simulink model "model8"  (R2014a)
settings: Solver=ode4  SolverMode=SingleTasking  StartTime=0.0  StopTime=200.0  FixedStep=.1  RelTol=1e-3
values from neighbouring files (symbols this model uses):
  K0 = diag([w^3,w^3,w^3.5])    [robot_mod_run.m]
  K1 = diag([2*w,2*w,4*w])    [robot_mod_run.m]
  k_ts = 0.29    [robot_mod_run.m]
  Kd = diag([5.4, 5.5, 3.8])    [robot_mod_run.m]
  Kp = diag([1, 1, 1])    [robot_mod_run.m]
  l_ts = .95    (= 0.95)    [robot_mod_run.m]
  qd1 = 1    [robot_mod_run.m]
  qd2 = 1    [robot_mod_run.m]
  qd3 = 1    [robot_mod_run.m]
  R_ts = .5    (= 0.5)    [robot_mod_run.m]
  time_gain_ts = .278    (= 0.278)    [robot_mod_run.m]
undefined symbols (not defined in the file or in its folder): forward_optim
libraries: aerolibutil x3
settings Model: Creator=Fu  LastModifiedBy=Fu
settings OptimizationCC: BlockReduction=off  BooleanDataType=off
settings DebuggingCC: SaveWithParameterizedLinksMsg=none  UnderspecifiedInitializationDetection=Classic  SignalResolutionControl=TryResolveAllWithWarning  SolverPrmCheckMsg=none
settings HardwareCC: TargetUnknown=on

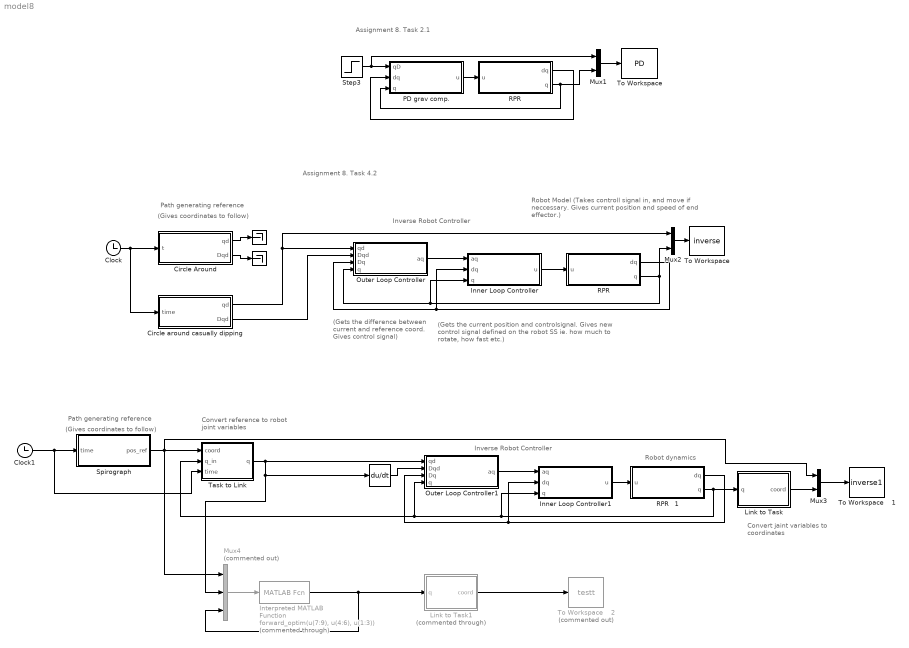
== system model8 ==
  note: Convert jaint variables
      | to coordinates
  note: Robot dynamics
  note: Convert reference to
      | robot joint variables
  note: (Gets the current position and controlsignal.
      | Gives new control signal defined on the robot SS
      | ie. how much to rotate, how fast etc.)
  note: (Gets the difference between
      |  current and reference coord.
      | Gives control signal)
  note: (Gives coordinates to follow)
  note: Robot Model
      | (Takes controll signal in, and move if neccessary.
      | Gives current position and speed of end effector.)
  note: Inverse Robot Controller
  note: Path generating reference
  note: Assignment 8. Task 4.2
  note: Assignment 8. Task 2.1
  note: Inverse Robot Controller
  note: (Gives coordinates to follow)
  note: Path generating reference
  " " : Derivative
  " " : Terminator
  "  " : Terminator
  Circle Around : Subsystem
  Circle around casually dipping : Subsystem
  Clock : Clock
  Clock1 : Clock
  Inner Loop Controller : Subsystem
  Inner Loop Controller1 : Subsystem
  Interpreted MATLAB Function : MATLABFcn  Commented=through  MATLABFcn=forward_optim(u(7:9), u(4:6), u(1:3))  OutputDimensions=3
  Link to Task : MATLAB Function  TreatAsAtomicUnit=on
  Link to Task1 : MATLAB Function  Commented=through  TreatAsAtomicUnit=on
  Mux1 : Mux  Inputs=2
  Mux2 : Mux  Inputs=2
  Mux3 : Mux  Inputs=2
  Mux4 : Mux  Commented=on  Inputs=3
  Outer Loop Controller : Subsystem
  Outer Loop Controller1 : Subsystem
  PD grav comp. : Subsystem
  RPR : Subsystem
  "RPR   " : Subsystem
  RPR   1 : Subsystem
  "Spirograph " : Subsystem
  Step3 : Step  Time=0  Before=[0;0;0]  After=[qd1;qd2;qd3]  SampleTime=0
  Task to Link : MATLAB Function  TreatAsAtomicUnit=on
  To Workspace : ToWorkspace  VariableName=PD  SaveFormat=Timeseries  SampleTime=-1
      settings: Save2DSignal=2-D array (concatenate along first dimension)
  "To Workspace    " : ToWorkspace  VariableName=inverse  SaveFormat=Timeseries  SampleTime=-1
      settings: Save2DSignal=2-D array (concatenate along first dimension)
  To Workspace    1 : ToWorkspace  VariableName=inverse1  SaveFormat=Timeseries  SampleTime=-1
      settings: Save2DSignal=2-D array (concatenate along first dimension)
  To Workspace    2 : ToWorkspace  Commented=on  VariableName=testt  SaveFormat=Timeseries  SampleTime=-1
      settings: Save2DSignal=2-D array (concatenate along first dimension)
  wires:
  PD grav comp./1(u) -> RPR/1(u)
  Step3/1 -> Mux1/1, PD grav comp./1(qD)
  RPR/2(q) -> Mux1/2, PD grav comp./3(q)
  RPR/1(dq) -> PD grav comp./2(dq)
  Inner Loop Controller/1(u) -> "RPR   "/1(u)
  "RPR   "/2(q) -> Mux2/2, Inner Loop Controller/3(q), Outer Loop Controller/4(q)
  "RPR   "/1(dq) -> Outer Loop Controller/3(Dq), Inner Loop Controller/2(dq)
  Outer Loop Controller/1(aq) -> Inner Loop Controller/1(aq)
  Clock/1 -> Circle around casually dipping/1(time), Circle Around/1(t)
  Mux1/1 -> To Workspace/1
  Mux2/1 -> "To Workspace    "/1
  Circle around casually dipping/1(qd) -> Outer Loop Controller/1(qd), Mux2/1
  Circle around casually dipping/2(Dqd) -> Outer Loop Controller/2(Dqd)
  Circle Around/1(qd) -> " "/1
  Circle Around/2(Dqd) -> "  "/1
  Inner Loop Controller1/1(u) -> RPR   1/1(u)
  RPR   1/2(q) -> Link to Task/1(q), Inner Loop Controller1/3(q), Outer Loop Controller1/4(q), Task to Link/2(q_in)
  RPR   1/1(dq) -> Outer Loop Controller1/3(Dq), Inner Loop Controller1/2(dq)
  Outer Loop Controller1/1(aq) -> Inner Loop Controller1/1(aq)
  Clock1/1 -> Task to Link/3(time), "Spirograph "/1(time)
  "Spirograph "/1(pos_ref) -> Mux4/1, Mux3/1, Task to Link/1(coord)
  Task to Link/1(q) -> Outer Loop Controller1/1(qd), " "/1, Mux4/2
  " "/1 -> Outer Loop Controller1/2(Dqd)
  Mux3/1 -> To Workspace    1/1
  Link to Task/1(coord) -> Mux3/2
  Mux4/1 -> Interpreted MATLAB Function/1
  Interpreted MATLAB Function/1 -> Mux4/3, Link to Task1/1(q)
  Link to Task1/1(coord) -> To Workspace    2/1

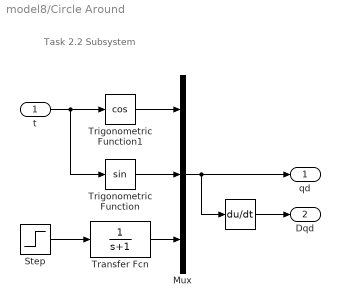
== system model8/Circle Around ==
  note: Task 2.2 Subsystem
  t : Inport
  " " : Derivative
  Mux : Mux  Inputs=3
  Step : Step  SampleTime=0
  Transfer Fcn : TransferFcn  Denominator=[1 1]
  Trigonometric Function : Trigonometry
  Trigonometric Function1 : Trigonometry  Operator=cos
  qd : Outport
  Dqd : Outport  Port=2
  wires:
  Mux/1 -> " "/1, qd/1
  t/1 -> Trigonometric Function/1, Trigonometric Function1/1
  Trigonometric Function1/1 -> Mux/1
  Trigonometric Function/1 -> Mux/2
  Step/1 -> Transfer Fcn/1
  Transfer Fcn/1 -> Mux/3
  " "/1 -> Dqd/1

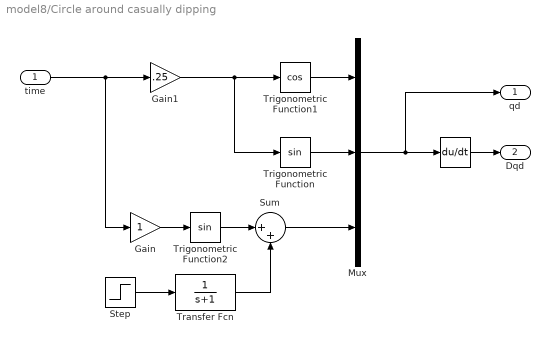
== system model8/Circle around casually dipping ==
  time : Inport
  " " : Derivative
  Gain : Gain
  Gain1 : Gain  Gain=.25
  Mux : Mux  Inputs=3
  Step : Step  SampleTime=0
  Sum : Sum  Inputs=|++
  Transfer Fcn : TransferFcn  Denominator=[1 1]
  Trigonometric Function : Trigonometry
  Trigonometric Function1 : Trigonometry  Operator=cos
  Trigonometric Function2 : Trigonometry
  qd : Outport
  Dqd : Outport  Port=2
  wires:
  Trigonometric Function1/1 -> Mux/1
  Trigonometric Function/1 -> Mux/2
  Mux/1 -> " "/1, qd/1
  " "/1 -> Dqd/1
  time/1 -> Gain1/1, Gain/1
  Step/1 -> Transfer Fcn/1
  Sum/1 -> Mux/3
  Transfer Fcn/1 -> Sum/2
  Gain/1 -> Trigonometric Function2/1
  Trigonometric Function2/1 -> Sum/1
  Gain1/1 -> Trigonometric Function1/1, Trigonometric Function/1

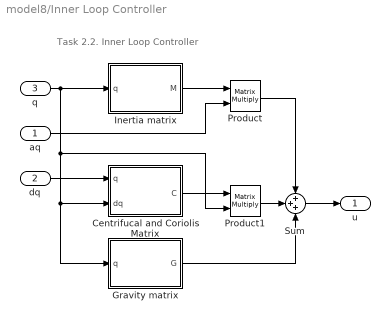
== system model8/Inner Loop Controller ==
  note: Task 2.2. Inner Loop Controller
  aq : Inport
  dq : Inport  Port=2
  q : Inport  Port=3
  Centrifucal and Coriolis Matrix : MATLAB Function  TreatAsAtomicUnit=on
  Gravity matrix : MATLAB Function  TreatAsAtomicUnit=on
  Inertia matrix : MATLAB Function  TreatAsAtomicUnit=on
  Product : Product  Multiplication=Matrix(*)
  Product1 : Product  Multiplication=Matrix(*)
  Sum : Sum  Inputs=+++
  u : Outport
  wires:
  Inertia matrix/1(M) -> Product/1
  aq/1 -> Product/2
  q/1 -> Inertia matrix/1(q), Centrifucal and Coriolis Matrix/2(dq), Gravity matrix/1(q), Product1/2
  Product/1 -> Sum/1
  dq/1 -> Centrifucal and Coriolis Matrix/1(q)
  Centrifucal and Coriolis Matrix/1(C) -> Product1/1
  Product1/1 -> Sum/2
  Gravity matrix/1(G) -> Sum/3
  Sum/1 -> u/1

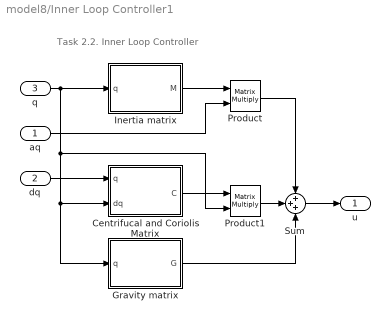
== system model8/Inner Loop Controller1 ==
  note: Task 2.2. Inner Loop Controller
  aq : Inport
  dq : Inport  Port=2
  q : Inport  Port=3
  Centrifucal and Coriolis Matrix : MATLAB Function  TreatAsAtomicUnit=on
  Gravity matrix : MATLAB Function  TreatAsAtomicUnit=on
  Inertia matrix : MATLAB Function  TreatAsAtomicUnit=on
  Product : Product  Multiplication=Matrix(*)
  Product1 : Product  Multiplication=Matrix(*)
  Sum : Sum  Inputs=+++
  u : Outport
  wires:
  Inertia matrix/1(M) -> Product/1
  aq/1 -> Product/2
  q/1 -> Inertia matrix/1(q), Centrifucal and Coriolis Matrix/2(dq), Gravity matrix/1(q), Product1/2
  Product/1 -> Sum/1
  dq/1 -> Centrifucal and Coriolis Matrix/1(q)
  Centrifucal and Coriolis Matrix/1(C) -> Product1/1
  Product1/1 -> Sum/2
  Gravity matrix/1(G) -> Sum/3
  Sum/1 -> u/1

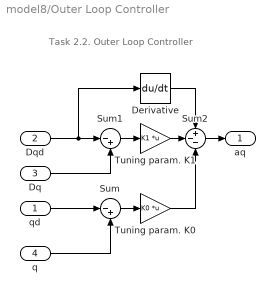
== system model8/Outer Loop Controller ==
  note: Task 2.2. Outer Loop Controller
  qd : Inport
  Dqd : Inport  Port=2
  Dq : Inport  Port=3
  q : Inport  Port=4
  Derivative : Derivative
  Sum : Sum  Inputs=|-+
  Sum1 : Sum  Inputs=|-+
  Sum2 : Sum  Inputs=+--
  Tuning param. K0 : Gain  Gain=K0  Multiplication=Matrix(K*u) (u vector)
  Tuning param. K1 : Gain  Gain=K1  Multiplication=Matrix(K*u) (u vector)
  aq : Outport
  wires:
  qd/1 -> Sum/1
  q/1 -> Sum/2
  Dq/1 -> Sum1/2
  Sum2/1 -> aq/1
  Derivative/1 -> Sum2/1
  Dqd/1 -> Derivative/1, Sum1/1
  Tuning param. K1/1 -> Sum2/2
  Sum1/1 -> Tuning param. K1/1
  Sum/1 -> Tuning param. K0/1
  Tuning param. K0/1 -> Sum2/3

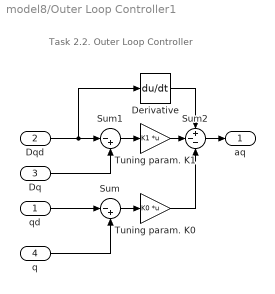
== system model8/Outer Loop Controller1 ==
  note: Task 2.2. Outer Loop Controller
  qd : Inport
  Dqd : Inport  Port=2
  Dq : Inport  Port=3
  q : Inport  Port=4
  Derivative : Derivative
  Sum : Sum  Inputs=|-+
  Sum1 : Sum  Inputs=|-+
  Sum2 : Sum  Inputs=+--
  Tuning param. K0 : Gain  Gain=K0  Multiplication=Matrix(K*u) (u vector)
  Tuning param. K1 : Gain  Gain=K1  Multiplication=Matrix(K*u) (u vector)
  aq : Outport
  wires:
  qd/1 -> Sum/1
  q/1 -> Sum/2
  Dq/1 -> Sum1/2
  Sum2/1 -> aq/1
  Derivative/1 -> Sum2/1
  Dqd/1 -> Derivative/1, Sum1/1
  Tuning param. K1/1 -> Sum2/2
  Sum1/1 -> Tuning param. K1/1
  Sum/1 -> Tuning param. K0/1
  Tuning param. K0/1 -> Sum2/3

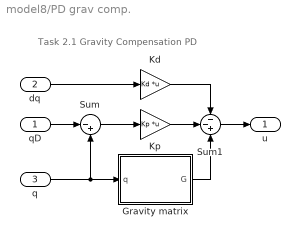
== system model8/PD grav comp. ==
  note: Task 2.1 Gravity Compensation PD
  qD : Inport
  dq : Inport  Port=2
  q : Inport  Port=3
  Gravity matrix : MATLAB Function  TreatAsAtomicUnit=on
  Kd : Gain  Gain=Kd  Multiplication=Matrix(K*u)
  Kp : Gain  Gain=Kp  Multiplication=Matrix(K*u)
  Sum : Sum  Inputs=|-+
  Sum1 : Sum  Inputs=--+
  u : Outport
  wires:
  Sum/1 -> Kp/1
  Kp/1 -> Sum1/2
  Kd/1 -> Sum1/1
  Gravity matrix/1(G) -> Sum1/3
  Sum1/1 -> u/1
  dq/1 -> Kd/1
  q/1 -> Gravity matrix/1(q), Sum/2
  qD/1 -> Sum/1

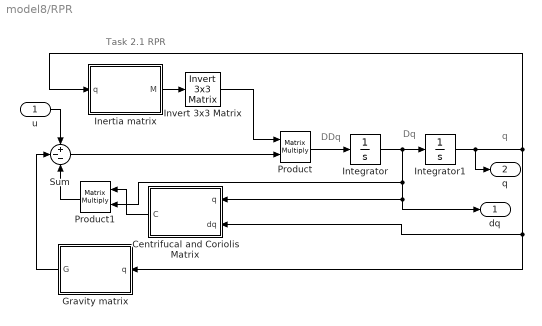
== system model8/RPR ==
  note: Task 2.1 RPR
  note: DDq
  note: q
  note: Dq
  u : Inport
  Centrifucal and Coriolis Matrix : MATLAB Function  TreatAsAtomicUnit=on
  Gravity matrix : MATLAB Function  TreatAsAtomicUnit=on
  Inertia matrix : MATLAB Function  TreatAsAtomicUnit=on
  Integrator : Integrator  InitialCondition=[0;0;0]
  Integrator1 : Integrator  InitialCondition=[1;0;0]
  Invert 3x3 Matrix : aerolibutil/Invert  3x3 Matrix
  Product : Product  Multiplication=Matrix(*)
  Product1 : Product  Multiplication=Matrix(*)
  Sum : Sum  Inputs=+--
  dq : Outport
  q : Outport  Port=2
  wires:
  Inertia matrix/1(M) -> Invert 3x3 Matrix/1
  Invert 3x3 Matrix/1 -> Product/1
  Product/1 -> Integrator/1
  Integrator/1 -> dq/1, Centrifucal and Coriolis Matrix/1(q), Product1/2, Integrator1/1
  Integrator1/1 -> Inertia matrix/1(q), Centrifucal and Coriolis Matrix/2(dq), Gravity matrix/1(q), q/1
  Sum/1 -> Product/2
  u/1 -> Sum/1
  Centrifucal and Coriolis Matrix/1(C) -> Product1/1
  Product1/1 -> Sum/3
  Gravity matrix/1(G) -> Sum/2

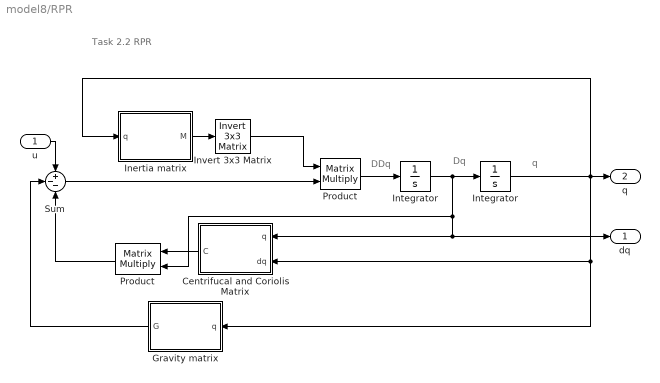
== system model8/RPR    ==
  note: Task 2.2 RPR
  note: DDq
  note: q
  note: Dq
  u : Inport
  Centrifucal and Coriolis Matrix : MATLAB Function  TreatAsAtomicUnit=on
  Gravity matrix : MATLAB Function  TreatAsAtomicUnit=on
  Inertia matrix : MATLAB Function  TreatAsAtomicUnit=on
  Integrator : Integrator  InitialCondition=[0;0;0]
  "Integrator " : Integrator  InitialCondition=[1;0;0]
  Invert 3x3 Matrix : aerolibutil/Invert  3x3 Matrix
  Product : Product  Multiplication=Matrix(*)
  "Product " : Product  Multiplication=Matrix(*)
  Sum : Sum  Inputs=+--
  dq : Outport
  q : Outport  Port=2
  wires:
  Inertia matrix/1(M) -> Invert 3x3 Matrix/1
  Invert 3x3 Matrix/1 -> Product/1
  Product/1 -> Integrator/1
  Integrator/1 -> Centrifucal and Coriolis Matrix/1(q), dq/1, "Product "/2, "Integrator "/1
  "Integrator "/1 -> Inertia matrix/1(q), q/1, Centrifucal and Coriolis Matrix/2(dq), Gravity matrix/1(q)
  Sum/1 -> Product/2
  u/1 -> Sum/1
  Centrifucal and Coriolis Matrix/1(C) -> "Product "/1
  "Product "/1 -> Sum/3
  Gravity matrix/1(G) -> Sum/2

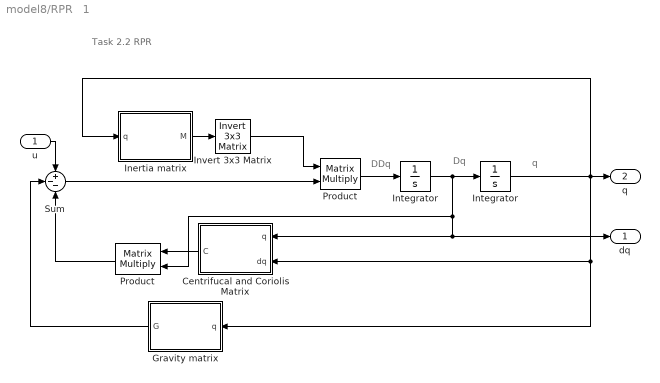
== system model8/RPR   1 ==
  note: Task 2.2 RPR
  note: DDq
  note: q
  note: Dq
  u : Inport
  Centrifucal and Coriolis Matrix : MATLAB Function  TreatAsAtomicUnit=on
  Gravity matrix : MATLAB Function  TreatAsAtomicUnit=on
  Inertia matrix : MATLAB Function  TreatAsAtomicUnit=on
  Integrator : Integrator  InitialCondition=[0;0;0]
  "Integrator " : Integrator  InitialCondition=[0;0;0]
  Invert 3x3 Matrix : aerolibutil/Invert  3x3 Matrix
  Product : Product  Multiplication=Matrix(*)
  "Product " : Product  Multiplication=Matrix(*)
  Sum : Sum  Inputs=+--
  dq : Outport
  q : Outport  Port=2
  wires:
  Inertia matrix/1(M) -> Invert 3x3 Matrix/1
  Invert 3x3 Matrix/1 -> Product/1
  Product/1 -> Integrator/1
  Integrator/1 -> Centrifucal and Coriolis Matrix/1(q), dq/1, "Product "/2, "Integrator "/1
  "Integrator "/1 -> Inertia matrix/1(q), q/1, Centrifucal and Coriolis Matrix/2(dq), Gravity matrix/1(q)
  Sum/1 -> Product/2
  u/1 -> Sum/1
  Centrifucal and Coriolis Matrix/1(C) -> "Product "/1
  "Product "/1 -> Sum/3
  Gravity matrix/1(G) -> Sum/2

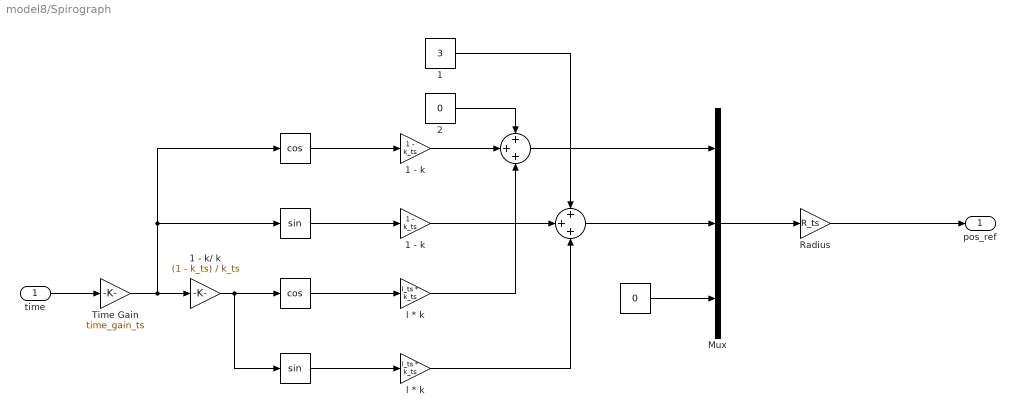
== system model8/Spirograph  ==
  time : Inport
  "    " : Constant  Value=0
  "     " : Trigonometry  Operator=cos
  "      " : Trigonometry
  "       " : Trigonometry  Operator=cos
  "        " : Trigonometry
  "         " : Sum  Inputs=+++
  "          " : Sum  Inputs=+++
  "    1" : Constant  Value=3
  "    2" : Constant  Value=0
  1 - k : Gain  Gain=1 - k_ts
  "1 - k " : Gain  Gain=1 - k_ts
  1 - k/ k : Gain  Gain=(1 - k_ts) / k_ts
  Mux : Mux  Inputs=3
  Radius : Gain  Gain=R_ts
  Time Gain : Gain  Gain=time_gain_ts
  l * k : Gain  Gain=l_ts * k_ts
  "l * k " : Gain  Gain=l_ts * k_ts
  pos_ref : Outport
  wires:
  Mux/1 -> Radius/1
  time/1 -> Time Gain/1
  1 - k/ k/1 -> "       "/1, "        "/1
  "     "/1 -> "1 - k "/1
  "      "/1 -> 1 - k/1
  "       "/1 -> l * k/1
  "        "/1 -> "l * k "/1
  Radius/1 -> pos_ref/1
  Time Gain/1 -> "     "/1, "      "/1, 1 - k/ k/1
  "    "/1 -> Mux/3
  "          "/1 -> Mux/2
  "         "/1 -> Mux/1
  "1 - k "/1 -> "         "/2
  l * k/1 -> "         "/3
  "l * k "/1 -> "          "/3
  1 - k/1 -> "          "/2
  "    1"/1 -> "          "/1
  "    2"/1 -> "         "/1

== matlab function model8/Inner Loop Controller1/Centrifucal and Coriolis Matrix ==
  data: q input; C output; dq input
function C = centriCori(q,dq)
%% Parameters
% Global variables in MATLAB if preferred (remove comments in that case)
% global m1 m2 m3;            % Masses
% global l1 l2 l3;            % Link lengths
% global lc1 lc2 lc3; 	      % Centers of mass
% global In1yy In2zz In3zz;   % Moment of inertia
% global gy;                  % Gravity force

% State variables
q1 = q(1);
q2 = q(2);
q3 = q(3);

dq1 = dq(1);
dq2 = dq(2);
dq3 = dq(3);

%syms q1 q2 q3 dq1 dq2 dq3;
m1 = 5; m2 = 5; m3 = 5;
l1 = 0.5; l2 = 0.5; l3 = 0.5;
lc1 = 0.5/2; lc2 = -0.5/2; lc3 = 0.5/2;
In1yy = 1/12*(m1*(l1)^2);
In2zz = 1/12*(m2*(l2)^2);
In3zz = 1/12*(m3*(l3)^2);

gy =9.81;

%% Matrices
% (8.21) Page 295 in book: M(q)*DDq + C(q,Dq)*Dq + G(q) = u
% Centrifugal and Coriolis matrix
C = [...
        (-0.2e1 * m3 * lc3 * cos(q1) * sin(q1 + q3) + 0.2e1 * m3 * lc3 * sin(q1) * cos(q1 + q3) + 0.2e1 * (m2 + m3) * q2 - 0.2e1 * m2 * lc2) * dq2 / 0.2e1 + (-0.2e1 * m3 * lc3 * cos(q1) * q2 * cos(q1 + q3) - 0.2e1 * m3 * lc3 * sin(q1) * q2 * sin(q1 + q3)) * dq3 / 0.2e1 (-0.2e1 * m3 * lc3 * cos(q1) * sin(q1 + q3) + 0.2e1 * m3 * lc3 * sin(q1) * cos(q1 + q3) + 0.2e1 * (m2 + m3) * q2 - 0.2e1 * m2 * lc2) * dq1 / 0.2e1 (-0.2e1 * m3 * lc3 * cos(q1) * q2 * cos(q1 + q3) - 0.2e1 * m3 * lc3 * sin(q1) * q2 * sin(q1 + q3)) * dq1 / 0.2e1 + (-m3 * lc3 * cos(q1) * q2 * cos(q1 + q3) - m3 * lc3 * sin(q1) * q2 * sin(q1 + q3)) * dq3; ...
        (-m3 * lc3 * sin(q1) * cos(q1 + q3) + m3 * lc3 * cos(q1) * sin(q1 + q3) - (m2 + m3) * q2 + m2 * lc2) * dq1 + (-0.2e1 * m3 * lc3 * sin(q1) * cos(q1 + q3) + 0.2e1 * m3 * lc3 * cos(q1) * sin(q1 + q3)) * dq3 / 0.2e1 0 (-0.2e1 * m3 * lc3 * sin(q1) * cos(q1 + q3) + 0.2e1 * m3 * lc3 * cos(q1) * sin(q1 + q3)) * dq1 / 0.2e1 + (-m3 * lc3 * sin(q1) * cos(q1 + q3) + m3 * lc3 * cos(q1) * sin(q1 + q3)) * dq3; 
        (m3 * lc3 * cos(q1) * q2 * cos(q1 + q3) + m3 * lc3 * sin(q1) * q2 * sin(q1 + q3)) * dq1 + (0.2e1 * m3 * lc3 * sin(q1) * cos(q1 + q3) - 0.2e1 * m3 * lc3 * cos(q1) * sin(q1 + q3)) * dq2 / 0.2e1 (0.2e1 * m3 * lc3 * sin(q1) * cos(q1 + q3) - 0.2e1 * m3 * lc3 * cos(q1) * sin(q1 + q3)) * dq1 / 0.2e1 0;...
     ];
end

== matlab function model8/Inner Loop Controller1/Gravity matrix ==
  data: q input; G output
function G = gravity(q)
% Global variables in MATLAB if preferred (remove comments in that case)
% global m1 m2 m3;            % Masses
% global l1 l2 l3;            % Link lengths
% global lc1 lc2 lc3; 	      % Centers of mass
% global In1yy In2zz In3zz;   % Moment of inertia
% global gy;                  % Gravity force

% State variables
q1 = q(1);
q2 = q(2);
q3 = q(3);

m1 = 5; m2 = 5; m3 = 5;
l1 = 0.5; l2 = 0.5; l3 = 0.5;
lc1 = 0.5/2; lc2 = -0.5/2; lc3 = 0.5/2;
In1yy = 1/12*(m1*(l1)^2);
In2zz = 1/12*(m2*(l2)^2);
In3zz = 1/12*(m3*(l3)^2);

gy = 9.81;

%% Matrices
% (8.21) Page 295 in book: M(q)*DDq + C(q,Dq)*Dq + G(q) = u
% Gravity vector
G = [(m3 * cos(q1 + q3) * lc3 + sin(q1) * q2 * m2 + sin(q1) * q2 * m3 + sin(q1) * lc1 * m1 - sin(q1) * m2 * lc2) * gy; -(m2 + m3) * cos(q1) * gy; m3 * cos(q1 + q3) * lc3 * gy;];

== matlab function model8/Inner Loop Controller/Centrifucal and Coriolis Matrix ==
  data: q input; C output; dq input
function C = centriCori(q,dq)
%% Parameters
% Global variables in MATLAB if preferred (remove comments in that case)
% global m1 m2 m3;            % Masses
% global l1 l2 l3;            % Link lengths
% global lc1 lc2 lc3; 	      % Centers of mass
% global In1yy In2zz In3zz;   % Moment of inertia
% global gy;                  % Gravity force

% State variables
q1 = q(1);
q2 = q(2);
q3 = q(3);

dq1 = dq(1);
dq2 = dq(2);
dq3 = dq(3);

%syms q1 q2 q3 dq1 dq2 dq3;
m1 = 5; m2 = 5; m3 = 5;
l1 = 0.5; l2 = 0.5; l3 = 0.5;
lc1 = 0.5/2; lc2 = -0.5/2; lc3 = 0.5/2;
In1yy = 1/12*(m1*(l1)^2);
In2zz = 1/12*(m2*(l2)^2);
In3zz = 1/12*(m3*(l3)^2);

gy =9.81;

%% Matrices
% (8.21) Page 295 in book: M(q)*DDq + C(q,Dq)*Dq + G(q) = u
% Centrifugal and Coriolis matrix
C = [...
        (-0.2e1 * m3 * lc3 * cos(q1) * sin(q1 + q3) + 0.2e1 * m3 * lc3 * sin(q1) * cos(q1 + q3) + 0.2e1 * (m2 + m3) * q2 - 0.2e1 * m2 * lc2) * dq2 / 0.2e1 + (-0.2e1 * m3 * lc3 * cos(q1) * q2 * cos(q1 + q3) - 0.2e1 * m3 * lc3 * sin(q1) * q2 * sin(q1 + q3)) * dq3 / 0.2e1 (-0.2e1 * m3 * lc3 * cos(q1) * sin(q1 + q3) + 0.2e1 * m3 * lc3 * sin(q1) * cos(q1 + q3) + 0.2e1 * (m2 + m3) * q2 - 0.2e1 * m2 * lc2) * dq1 / 0.2e1 (-0.2e1 * m3 * lc3 * cos(q1) * q2 * cos(q1 + q3) - 0.2e1 * m3 * lc3 * sin(q1) * q2 * sin(q1 + q3)) * dq1 / 0.2e1 + (-m3 * lc3 * cos(q1) * q2 * cos(q1 + q3) - m3 * lc3 * sin(q1) * q2 * sin(q1 + q3)) * dq3; ...
        (-m3 * lc3 * sin(q1) * cos(q1 + q3) + m3 * lc3 * cos(q1) * sin(q1 + q3) - (m2 + m3) * q2 + m2 * lc2) * dq1 + (-0.2e1 * m3 * lc3 * sin(q1) * cos(q1 + q3) + 0.2e1 * m3 * lc3 * cos(q1) * sin(q1 + q3)) * dq3 / 0.2e1 0 (-0.2e1 * m3 * lc3 * sin(q1) * cos(q1 + q3) + 0.2e1 * m3 * lc3 * cos(q1) * sin(q1 + q3)) * dq1 / 0.2e1 + (-m3 * lc3 * sin(q1) * cos(q1 + q3) + m3 * lc3 * cos(q1) * sin(q1 + q3)) * dq3; 
        (m3 * lc3 * cos(q1) * q2 * cos(q1 + q3) + m3 * lc3 * sin(q1) * q2 * sin(q1 + q3)) * dq1 + (0.2e1 * m3 * lc3 * sin(q1) * cos(q1 + q3) - 0.2e1 * m3 * lc3 * cos(q1) * sin(q1 + q3)) * dq2 / 0.2e1 (0.2e1 * m3 * lc3 * sin(q1) * cos(q1 + q3) - 0.2e1 * m3 * lc3 * cos(q1) * sin(q1 + q3)) * dq1 / 0.2e1 0;...
     ];
end

== matlab function model8/Inner Loop Controller1/Inertia matrix ==
  data: q input; M output
function M = inertia(q)
%% Parameters
% Global variables in MATLAB if preferred (remove comments in that case)
% global m1 m2 m3;            % Masses
% global l1 l2 l3;            % Link lengths
% global lc1 lc2 lc3; 	      % Centers of mass
% global In1yy In2zz In3zz;   % Moment of inertia
% global gy;                  % Gravity force

% State variables
q1 = q(1);
q2 = q(2);
q3 = q(3);

%dq1 = dq(1);
%dq2 = dq(2);
%dq3 = dq(3);

m1 = 5; m2 = 5; m3 = 5;
l1 = 0.5; l2 = 0.5; l3 = 0.5;
lc1 = 0.5/2; lc2 = -0.5/2; lc3 = 0.5/2;
In1yy = 1/12*(m1*(l1)^2);
In2zz = 1/12*(m2*(l2)^2);
In3zz = 1/12*(m3*(l3)^2);
gy = 9.81;

%% Matrices
% (8.21) Page 295 in book: M(q)*DDq + C(q,Dq)*Dq + G(q) = u
M = [   ...
        0.2e1 * m3 * lc3 * cos(q1 + q3) * sin(q1) * q2 - 0.2e1 * m3 * lc3 * sin(q1 + q3) * cos(q1) * q2 + (m2 + m3) * q2 ^ 2 - 0.2e1 * m2 * lc2 * q2 + m1 * lc1 ^ 2 + In1yy + m2 * lc2 ^ 2 + In3zz + In2zz + m3 * lc3 ^ 2 -m3 * lc3 * sin(q1) * sin(q1 + q3) - m3 * lc3 * cos(q1) * cos(q1 + q3) m3 * lc3 ^ 2 - m3 * lc3 * sin(q1 + q3) * cos(q1) * q2 + m3 * lc3 * cos(q1 + q3) * sin(q1) * q2 + In3zz; ...
        -m3 * lc3 * sin(q1) * sin(q1 + q3) - m3 * lc3 * cos(q1) * cos(q1 + q3) m2 + m3 -m3 * lc3 * sin(q1) * sin(q1 + q3) - m3 * lc3 * cos(q1) * cos(q1 + q3); ...
        m3 * lc3 ^ 2 - m3 * lc3 * sin(q1 + q3) * cos(q1) * q2 + m3 * lc3 * cos(q1 + q3) * sin(q1) * q2 + In3zz -m3 * lc3 * sin(q1) * sin(q1 + q3) - m3 * lc3 * cos(q1) * cos(q1 + q3) m3 * lc3 ^ 2 + In3zz; ...
    ];

end

== matlab function model8/RPR/Centrifucal and Coriolis Matrix ==
  data: q input; C output; dq input
function C = centriCori(q,dq)
%% Parameters
% Global variables in MATLAB if preferred (remove comments in that case)
% global m1 m2 m3;            % Masses
% global l1 l2 l3;            % Link lengths
% global lc1 lc2 lc3; 	      % Centers of mass
% global In1yy In2zz In3zz;   % Moment of inertia
q1 = q(1);
q2 = q(2);
q3 = q(3);
dq1 = dq(1);
dq2 = dq(2);
dq3 = dq(3);

%syms q1 q2 q3 dq1 dq2 dq3;
m1 = 5; m2 = 5; m3 = 5;
l1 = 0.5; l2 = 0.5; l3 = 0.5;
lc1 = 0.5/2; lc2 = -0.5/2; lc3 = 0.5/2;
In1yy = 1/12*(m1*(l1)^2);
In2zz = 1/12*(m2*(l2)^2);
In3zz = 1/12*(m3*(l3)^2);
gy =9.81;
%% Matrices
% (8.21) Page 295 in book: M(q)*DDq + C(q,Dq)*Dq + G(q) = u
% gy = 9.81
% Gravity vector
%G = [(m3 * cos(q1 + q3) * lc3 + sin(q1) * q2 * m2 + sin(q1) * q2 * m3 + sin(q1) * lc1 * m1 - sin(q1) * m2 * lc2) * gy; -(m2 + m3) * cos(q1) * gy; m3 * cos(q1 + q3) * lc3 * gy;];
% Centrifugal and Coriolis matrix
C = [(-0.2e1 * m3 * lc3 * cos(q1) * sin(q1 + q3) + 0.2e1 * m3 * lc3 * sin(q1) * cos(q1 + q3) + 0.2e1 * (m2 + m3) * q2 - 0.2e1 * m2 * lc2) * dq2 / 0.2e1 + (-0.2e1 * m3 * lc3 * cos(q1) * q2 * cos(q1 + q3) - 0.2e1 * m3 * lc3 * sin(q1) * q2 * sin(q1 + q3)) * dq3 / 0.2e1 (-0.2e1 * m3 * lc3 * cos(q1) * sin(q1 + q3) + 0.2e1 * m3 * lc3 * sin(q1) * cos(q1 + q3) + 0.2e1 * (m2 + m3) * q2 - 0.2e1 * m2 * lc2) * dq1 / 0.2e1 (-0.2e1 * m3 * lc3 * cos(q1) * q2 * cos(q1 + q3) - 0.2e1 * m3 * lc3 * sin(q1) * q2 * sin(q1 + q3)) * dq1 / 0.2e1 + (-m3 * lc3 * cos(q1) * q2 * cos(q1 + q3) - m3 * lc3 * sin(q1) * q2 * sin(q1 + q3)) * dq3; (-m3 * lc3 * sin(q1) * cos(q1 + q3) + m3 * lc3 * cos(q1) * sin(q1 + q3) - (m2 + m3) * q2 + m2 * lc2) * dq1 + (-0.2e1 * m3 * lc3 * sin(q1) * cos(q1 + q3) + 0.2e1 * m3 * lc3 * cos(q1) * sin(q1 + q3)) * dq3 / 0.2e1 0 (-0.2e1 * m3 * lc3 * sin(q1) * cos(q1 + q3) + 0.2e1 * m3 * lc3 * cos(q1) * sin(q1 + q3)) * dq1 / 0.2e1 + (-m3 * lc3 * sin(q1) * cos(q1 + q3) + m3 * lc3 * cos(q1) * sin(q1 + q3)) * dq3; (m3 * lc3 * cos(q1) * q2 * cos(q1 + q3) + m3 * lc3 * sin(q1) * q2 * sin(q1 + q3)) * dq1 + (0.2e1 * m3 * lc3 * sin(q1) * cos(q1 + q3) - 0.2e1 * m3 * lc3 * cos(q1) * sin(q1 + q3)) * dq2 / 0.2e1 (0.2e1 * m3 * lc3 * sin(q1) * cos(q1 + q3) - 0.2e1 * m3 * lc3 * cos(q1) * sin(q1 + q3)) * dq1 / 0.2e1 0;];
% Inertia matrix
%M = [0.2e1 * m3 * lc3 * cos(q1 + q3) * sin(q1) * q2 - 0.2e1 * m3 * lc3 * sin(q1 + q3) * cos(q1) * q2 + (m2 + m3) * q2 ^ 2 - 0.2e1 * m2 * lc2 * q2 + m1 * lc1 ^ 2 + In1yy + m2 * lc2 ^ 2 + In3zz + In2zz + m3 * lc3 ^ 2 -m3 * lc3 * sin(q1) * sin(q1 + q3) - m3 * lc3 * cos(q1) * cos(q1 + q3) m3 * lc3 ^ 2 - m3 * lc3 * sin(q1 + q3) * cos(q1) * q2 + m3 * lc3 * cos(q1 + q3) * sin(q1) * q2 + In3zz; -m3 * lc3 * sin(q1) * sin(q1 + q3) - m3 * lc3 * cos(q1) * cos(q1 + q3) m2 + m3 -m3 * lc3 * sin(q1) * sin(q1 + q3) - m3 * lc3 * cos(q1) * cos(q1 + q3); m3 * lc3 ^ 2 - m3 * lc3 * sin(q1 + q3) * cos(q1) * q2 + m3 * lc3 * cos(q1 + q3) * sin(q1) * q2 + In3zz -m3 * lc3 * sin(q1) * sin(q1 + q3) - m3 * lc3 * cos(q1) * cos(q1 + q3) m3 * lc3 ^ 2 + In3zz;];
end

== matlab function model8/PD grav comp./Gravity matrix ==
  data: q input; G output
function G = gravity(q)
%syms q1 q2 q3 dq1 dq2 dq3;
q1 = q(1);
q2 = q(2);
q3 = q(3);

m1 = 5; m2 = 5; m3 = 5;
l1 = 0.5; l2 = 0.5; l3 = 0.5;
lc1 = 0.5/2; lc2 = -0.5/2; lc3 = 0.5/2;
In1yy = 1/12*(m1*(l1)^2);
In2zz = 1/12*(m2*(l2)^2);
In3zz = 1/12*(m3*(l3)^2);
gy = 9.81;
%% Matrices
% (8.21) Page 295 in book: M(q)*DDq + C(q,Dq)*Dq + G(q) = u
gy = 9.81;
% Gravity vector
G = [(m3 * cos(q1 + q3) * lc3 + sin(q1) * q2 * m2 + sin(q1) * q2 * m3 + sin(q1) * lc1 * m1 - sin(q1) * m2 * lc2) * gy; -(m2 + m3) * cos(q1) * gy; m3 * cos(q1 + q3) * lc3 * gy;];

== matlab function model8/RPR/Gravity matrix ==
  data: q input; G output
function G = gravity(q)
%syms q1 q2 q3 dq1 dq2 dq3;
q1 = q(1);
q2 = q(2);
q3 = q(3);

m1 = 5; m2 = 5; m3 = 5;
l1 = 0.5; l2 = 0.5; l3 = 0.5;
lc1 = 0.5/2; lc2 = -0.5/2; lc3 = 0.5/2;
In1yy = 1/12*(m1*(l1)^2);
In2zz = 1/12*(m2*(l2)^2);
In3zz = 1/12*(m3*(l3)^2);
gy = 9.81;

%% Matrices
% (8.21) Page 295 in book: M(q)*DDq + C(q,Dq)*Dq + G(q) = u
% Gravity vector
G = [(m3 * cos(q1 + q3) * lc3 + sin(q1) * q2 * m2 + sin(q1) * q2 * m3 + sin(q1) * lc1 * m1 - sin(q1) * m2 * lc2) * gy; -(m2 + m3) * cos(q1) * gy; m3 * cos(q1 + q3) * lc3 * gy;];

== matlab function model8/RPR/Inertia matrix ==
  data: q input; M output
function M = inertia(q)
%% Parameters
% Global variables in MATLAB if preferred (remove comments in that case)
% global m1 m2 m3;            % Masses
% global l1 l2 l3;            % Link lengths
% global lc1 lc2 lc3; 	      % Centers of mass
% global In1yy In2zz In3zz;   % Moment of inertia
q1 = q(1);
q2 = q(2);
q3 = q(3);
%dq1 = dq(1);
%dq2 = dq(2);
%dq3 = dq(3);

%syms q1 q2 q3 dq1 dq2 dq3;
m1 = 5; m2 = 5; m3 = 5;
l1 = 0.5; l2 = 0.5; l3 = 0.5;
lc1 = 0.5/2; lc2 = -0.5/2; lc3 = 0.5/2;
In1yy = 1/12*(m1*(l1)^2);
In2zz = 1/12*(m2*(l2)^2);
In3zz = 1/12*(m3*(l3)^2);
gy =9.81;
%% Matrices
% (8.21) Page 295 in book: M(q)*DDq + C(q,Dq)*Dq + G(q) = u
% gy = 9.81
% Gravity vector
%G = [(m3 * cos(q1 + q3) * lc3 + sin(q1) * q2 * m2 + sin(q1) * q2 * m3 + sin(q1) * lc1 * m1 - sin(q1) * m2 * lc2) * gy; -(m2 + m3) * cos(q1) * gy; m3 * cos(q1 + q3) * lc3 * gy;];
% Centrifugal and Coriolis matrix
%C = [(-0.2e1 * m3 * lc3 * cos(q1) * sin(q1 + q3) + 0.2e1 * m3 * lc3 * sin(q1) * cos(q1 + q3) + 0.2e1 * (m2 + m3) * q2 - 0.2e1 * m2 * lc2) * dq2 / 0.2e1 + (-0.2e1 * m3 * lc3 * cos(q1) * q2 * cos(q1 + q3) - 0.2e1 * m3 * lc3 * sin(q1) * q2 * sin(q1 + q3)) * dq3 / 0.2e1 (-0.2e1 * m3 * lc3 * cos(q1) * sin(q1 + q3) + 0.2e1 * m3 * lc3 * sin(q1) * cos(q1 + q3) + 0.2e1 * (m2 + m3) * q2 - 0.2e1 * m2 * lc2) * dq1 / 0.2e1 (-0.2e1 * m3 * lc3 * cos(q1) * q2 * cos(q1 + q3) - 0.2e1 * m3 * lc3 * sin(q1) * q2 * sin(q1 + q3)) * dq1 / 0.2e1 + (-m3 * lc3 * cos(q1) * q2 * cos(q1 + q3) - m3 * lc3 * sin(q1) * q2 * sin(q1 + q3)) * dq3; (-m3 * lc3 * sin(q1) * cos(q1 + q3) + m3 * lc3 * cos(q1) * sin(q1 + q3) - (m2 + m3) * q2 + m2 * lc2) * dq1 + (-0.2e1 * m3 * lc3 * sin(q1) * cos(q1 + q3) + 0.2e1 * m3 * lc3 * cos(q1) * sin(q1 + q3)) * dq3 / 0.2e1 0 (-0.2e1 * m3 * lc3 * sin(q1) * cos(q1 + q3) + 0.2e1 * m3 * lc3 * cos(q1) * sin(q1 + q3)) * dq1 / 0.2e1 + (-m3 * lc3 * sin(q1) * cos(q1 + q3) + m3 * lc3 * cos(q1) * sin(q1 + q3)) * dq3; (m3 * lc3 * cos(q1) * q2 * cos(q1 + q3) + m3 * lc3 * sin(q1) * q2 * sin(q1 + q3)) * dq1 + (0.2e1 * m3 * lc3 * sin(q1) * cos(q1 + q3) - 0.2e1 * m3 * lc3 * cos(q1) * sin(q1 + q3)) * dq2 / 0.2e1 (0.2e1 * m3 * lc3 * sin(q1) * cos(q1 + q3) - 0.2e1 * m3 * lc3 * cos(q1) * sin(q1 + q3)) * dq1 / 0.2e1 0;];
% Inertia matrix
M = [0.2e1 * m3 * lc3 * cos(q1 + q3) * sin(q1) * q2 - 0.2e1 * m3 * lc3 * sin(q1 + q3) * cos(q1) * q2 + (m2 + m3) * q2 ^ 2 - 0.2e1 * m2 * lc2 * q2 + m1 * lc1 ^ 2 + In1yy + m2 * lc2 ^ 2 + In3zz + In2zz + m3 * lc3 ^ 2 -m3 * lc3 * sin(q1) * sin(q1 + q3) - m3 * lc3 * cos(q1) * cos(q1 + q3) m3 * lc3 ^ 2 - m3 * lc3 * sin(q1 + q3) * cos(q1) * q2 + m3 * lc3 * cos(q1 + q3) * sin(q1) * q2 + In3zz; -m3 * lc3 * sin(q1) * sin(q1 + q3) - m3 * lc3 * cos(q1) * cos(q1 + q3) m2 + m3 -m3 * lc3 * sin(q1) * sin(q1 + q3) - m3 * lc3 * cos(q1) * cos(q1 + q3); m3 * lc3 ^ 2 - m3 * lc3 * sin(q1 + q3) * cos(q1) * q2 + m3 * lc3 * cos(q1 + q3) * sin(q1) * q2 + In3zz -m3 * lc3 * sin(q1) * sin(q1 + q3) - m3 * lc3 * cos(q1) * cos(q1 + q3) m3 * lc3 ^ 2 + In3zz;];

end

== matlab function model8/Inner Loop Controller/Gravity matrix ==
  data: q input; G output
function G = gravity(q)
% Global variables in MATLAB if preferred (remove comments in that case)
% global m1 m2 m3;            % Masses
% global l1 l2 l3;            % Link lengths
% global lc1 lc2 lc3; 	      % Centers of mass
% global In1yy In2zz In3zz;   % Moment of inertia
% global gy;                  % Gravity force

% State variables
q1 = q(1);
q2 = q(2);
q3 = q(3);

m1 = 5; m2 = 5; m3 = 5;
l1 = 0.5; l2 = 0.5; l3 = 0.5;
lc1 = 0.5/2; lc2 = -0.5/2; lc3 = 0.5/2;
In1yy = 1/12*(m1*(l1)^2);
In2zz = 1/12*(m2*(l2)^2);
In3zz = 1/12*(m3*(l3)^2);

gy = 9.81;

%% Matrices
% (8.21) Page 295 in book: M(q)*DDq + C(q,Dq)*Dq + G(q) = u
% Gravity vector
G = [(m3 * cos(q1 + q3) * lc3 + sin(q1) * q2 * m2 + sin(q1) * q2 * m3 + sin(q1) * lc1 * m1 - sin(q1) * m2 * lc2) * gy; -(m2 + m3) * cos(q1) * gy; m3 * cos(q1 + q3) * lc3 * gy;];

== matlab function model8/Inner Loop Controller/Inertia matrix ==
  data: q input; M output
function M = inertia(q)
%% Parameters
% Global variables in MATLAB if preferred (remove comments in that case)
% global m1 m2 m3;            % Masses
% global l1 l2 l3;            % Link lengths
% global lc1 lc2 lc3; 	      % Centers of mass
% global In1yy In2zz In3zz;   % Moment of inertia
% global gy;                  % Gravity force

% State variables
q1 = q(1);
q2 = q(2);
q3 = q(3);

%dq1 = dq(1);
%dq2 = dq(2);
%dq3 = dq(3);

m1 = 5; m2 = 5; m3 = 5;
l1 = 0.5; l2 = 0.5; l3 = 0.5;
lc1 = 0.5/2; lc2 = -0.5/2; lc3 = 0.5/2;
In1yy = 1/12*(m1*(l1)^2);
In2zz = 1/12*(m2*(l2)^2);
In3zz = 1/12*(m3*(l3)^2);
gy = 9.81;

%% Matrices
% (8.21) Page 295 in book: M(q)*DDq + C(q,Dq)*Dq + G(q) = u
M = [   ...
        0.2e1 * m3 * lc3 * cos(q1 + q3) * sin(q1) * q2 - 0.2e1 * m3 * lc3 * sin(q1 + q3) * cos(q1) * q2 + (m2 + m3) * q2 ^ 2 - 0.2e1 * m2 * lc2 * q2 + m1 * lc1 ^ 2 + In1yy + m2 * lc2 ^ 2 + In3zz + In2zz + m3 * lc3 ^ 2 -m3 * lc3 * sin(q1) * sin(q1 + q3) - m3 * lc3 * cos(q1) * cos(q1 + q3) m3 * lc3 ^ 2 - m3 * lc3 * sin(q1 + q3) * cos(q1) * q2 + m3 * lc3 * cos(q1 + q3) * sin(q1) * q2 + In3zz; ...
        -m3 * lc3 * sin(q1) * sin(q1 + q3) - m3 * lc3 * cos(q1) * cos(q1 + q3) m2 + m3 -m3 * lc3 * sin(q1) * sin(q1 + q3) - m3 * lc3 * cos(q1) * cos(q1 + q3); ...
        m3 * lc3 ^ 2 - m3 * lc3 * sin(q1 + q3) * cos(q1) * q2 + m3 * lc3 * cos(q1 + q3) * sin(q1) * q2 + In3zz -m3 * lc3 * sin(q1) * sin(q1 + q3) - m3 * lc3 * cos(q1) * cos(q1 + q3) m3 * lc3 ^ 2 + In3zz; ...
    ];

end

== matlab function model8/RPR   /Centrifucal and Coriolis Matrix ==
  data: q input; C output; dq input
function C = centriCori(q,dq)
%% Parameters
% Global variables in MATLAB if preferred (remove comments in that case)
% global m1 m2 m3;            % Masses
% global l1 l2 l3;            % Link lengths
% global lc1 lc2 lc3; 	      % Centers of mass
% global In1yy In2zz In3zz;   % Moment of inertia
q1 = q(1);
q2 = q(2);
q3 = q(3);
dq1 = dq(1);
dq2 = dq(2);
dq3 = dq(3);

%syms q1 q2 q3 dq1 dq2 dq3;
m1 = 5; m2 = 5; m3 = 5;
l1 = 0.5; l2 = 0.5; l3 = 0.5;
lc1 = 0.5/2; lc2 = -0.5/2; lc3 = 0.5/2;
In1yy = 1/12*(m1*(l1)^2);
In2zz = 1/12*(m2*(l2)^2);
In3zz = 1/12*(m3*(l3)^2);
gy =9.81;
%% Matrices
% (8.21) Page 295 in book: M(q)*DDq + C(q,Dq)*Dq + G(q) = u
% gy = 9.81
% Gravity vector
%G = [(m3 * cos(q1 + q3) * lc3 + sin(q1) * q2 * m2 + sin(q1) * q2 * m3 + sin(q1) * lc1 * m1 - sin(q1) * m2 * lc2) * gy; -(m2 + m3) * cos(q1) * gy; m3 * cos(q1 + q3) * lc3 * gy;];
% Centrifugal and Coriolis matrix
C = [(-0.2e1 * m3 * lc3 * cos(q1) * sin(q1 + q3) + 0.2e1 * m3 * lc3 * sin(q1) * cos(q1 + q3) + 0.2e1 * (m2 + m3) * q2 - 0.2e1 * m2 * lc2) * dq2 / 0.2e1 + (-0.2e1 * m3 * lc3 * cos(q1) * q2 * cos(q1 + q3) - 0.2e1 * m3 * lc3 * sin(q1) * q2 * sin(q1 + q3)) * dq3 / 0.2e1 (-0.2e1 * m3 * lc3 * cos(q1) * sin(q1 + q3) + 0.2e1 * m3 * lc3 * sin(q1) * cos(q1 + q3) + 0.2e1 * (m2 + m3) * q2 - 0.2e1 * m2 * lc2) * dq1 / 0.2e1 (-0.2e1 * m3 * lc3 * cos(q1) * q2 * cos(q1 + q3) - 0.2e1 * m3 * lc3 * sin(q1) * q2 * sin(q1 + q3)) * dq1 / 0.2e1 + (-m3 * lc3 * cos(q1) * q2 * cos(q1 + q3) - m3 * lc3 * sin(q1) * q2 * sin(q1 + q3)) * dq3; (-m3 * lc3 * sin(q1) * cos(q1 + q3) + m3 * lc3 * cos(q1) * sin(q1 + q3) - (m2 + m3) * q2 + m2 * lc2) * dq1 + (-0.2e1 * m3 * lc3 * sin(q1) * cos(q1 + q3) + 0.2e1 * m3 * lc3 * cos(q1) * sin(q1 + q3)) * dq3 / 0.2e1 0 (-0.2e1 * m3 * lc3 * sin(q1) * cos(q1 + q3) + 0.2e1 * m3 * lc3 * cos(q1) * sin(q1 + q3)) * dq1 / 0.2e1 + (-m3 * lc3 * sin(q1) * cos(q1 + q3) + m3 * lc3 * cos(q1) * sin(q1 + q3)) * dq3; (m3 * lc3 * cos(q1) * q2 * cos(q1 + q3) + m3 * lc3 * sin(q1) * q2 * sin(q1 + q3)) * dq1 + (0.2e1 * m3 * lc3 * sin(q1) * cos(q1 + q3) - 0.2e1 * m3 * lc3 * cos(q1) * sin(q1 + q3)) * dq2 / 0.2e1 (0.2e1 * m3 * lc3 * sin(q1) * cos(q1 + q3) - 0.2e1 * m3 * lc3 * cos(q1) * sin(q1 + q3)) * dq1 / 0.2e1 0;];
% Inertia matrix
%M = [0.2e1 * m3 * lc3 * cos(q1 + q3) * sin(q1) * q2 - 0.2e1 * m3 * lc3 * sin(q1 + q3) * cos(q1) * q2 + (m2 + m3) * q2 ^ 2 - 0.2e1 * m2 * lc2 * q2 + m1 * lc1 ^ 2 + In1yy + m2 * lc2 ^ 2 + In3zz + In2zz + m3 * lc3 ^ 2 -m3 * lc3 * sin(q1) * sin(q1 + q3) - m3 * lc3 * cos(q1) * cos(q1 + q3) m3 * lc3 ^ 2 - m3 * lc3 * sin(q1 + q3) * cos(q1) * q2 + m3 * lc3 * cos(q1 + q3) * sin(q1) * q2 + In3zz; -m3 * lc3 * sin(q1) * sin(q1 + q3) - m3 * lc3 * cos(q1) * cos(q1 + q3) m2 + m3 -m3 * lc3 * sin(q1) * sin(q1 + q3) - m3 * lc3 * cos(q1) * cos(q1 + q3); m3 * lc3 ^ 2 - m3 * lc3 * sin(q1 + q3) * cos(q1) * q2 + m3 * lc3 * cos(q1 + q3) * sin(q1) * q2 + In3zz -m3 * lc3 * sin(q1) * sin(q1 + q3) - m3 * lc3 * cos(q1) * cos(q1 + q3) m3 * lc3 ^ 2 + In3zz;];
end

== matlab function model8/RPR   /Gravity matrix ==
  data: q input; G output
function G = gravity(q)
%syms q1 q2 q3 dq1 dq2 dq3;
q1 = q(1);
q2 = q(2);
q3 = q(3);

m1 = 5; m2 = 5; m3 = 5;
l1 = 0.5; l2 = 0.5; l3 = 0.5;
lc1 = 0.5/2; lc2 = -0.5/2; lc3 = 0.5/2;
In1yy = 1/12*(m1*(l1)^2);
In2zz = 1/12*(m2*(l2)^2);
In3zz = 1/12*(m3*(l3)^2);
gy = 9.81;
%% Matrices
% (8.21) Page 295 in book: M(q)*DDq + C(q,Dq)*Dq + G(q) = u
% Gravity vector
G = [(m3 * cos(q1 + q3) * lc3 + sin(q1) * q2 * m2 + sin(q1) * q2 * m3 + sin(q1) * lc1 * m1 - sin(q1) * m2 * lc2) * gy; -(m2 + m3) * cos(q1) * gy; m3 * cos(q1 + q3) * lc3 * gy;];

== matlab function model8/RPR   /Inertia matrix ==
  data: q input; M output
function M = inertia(q)
%% Parameters
% Global variables in MATLAB if preferred (remove comments in that case)
% global m1 m2 m3;            % Masses
% global l1 l2 l3;            % Link lengths
% global lc1 lc2 lc3; 	      % Centers of mass
% global In1yy In2zz In3zz;   % Moment of inertia
q1 = q(1);
q2 = q(2);
q3 = q(3);
%dq1 = dq(1);
%dq2 = dq(2);
%dq3 = dq(3);

%syms q1 q2 q3 dq1 dq2 dq3;
m1 = 5; m2 = 5; m3 = 5;
l1 = 0.5; l2 = 0.5; l3 = 0.5;
lc1 = 0.5/2; lc2 = -0.5/2; lc3 = 0.5/2;
In1yy = 1/12*(m1*(l1)^2);
In2zz = 1/12*(m2*(l2)^2);
In3zz = 1/12*(m3*(l3)^2);
gy =9.81;
%% Matrices
% (8.21) Page 295 in book: M(q)*DDq + C(q,Dq)*Dq + G(q) = u
% gy = 9.81
% Gravity vector
%G = [(m3 * cos(q1 + q3) * lc3 + sin(q1) * q2 * m2 + sin(q1) * q2 * m3 + sin(q1) * lc1 * m1 - sin(q1) * m2 * lc2) * gy; -(m2 + m3) * cos(q1) * gy; m3 * cos(q1 + q3) * lc3 * gy;];
% Centrifugal and Coriolis matrix
%C = [(-0.2e1 * m3 * lc3 * cos(q1) * sin(q1 + q3) + 0.2e1 * m3 * lc3 * sin(q1) * cos(q1 + q3) + 0.2e1 * (m2 + m3) * q2 - 0.2e1 * m2 * lc2) * dq2 / 0.2e1 + (-0.2e1 * m3 * lc3 * cos(q1) * q2 * cos(q1 + q3) - 0.2e1 * m3 * lc3 * sin(q1) * q2 * sin(q1 + q3)) * dq3 / 0.2e1 (-0.2e1 * m3 * lc3 * cos(q1) * sin(q1 + q3) + 0.2e1 * m3 * lc3 * sin(q1) * cos(q1 + q3) + 0.2e1 * (m2 + m3) * q2 - 0.2e1 * m2 * lc2) * dq1 / 0.2e1 (-0.2e1 * m3 * lc3 * cos(q1) * q2 * cos(q1 + q3) - 0.2e1 * m3 * lc3 * sin(q1) * q2 * sin(q1 + q3)) * dq1 / 0.2e1 + (-m3 * lc3 * cos(q1) * q2 * cos(q1 + q3) - m3 * lc3 * sin(q1) * q2 * sin(q1 + q3)) * dq3; (-m3 * lc3 * sin(q1) * cos(q1 + q3) + m3 * lc3 * cos(q1) * sin(q1 + q3) - (m2 + m3) * q2 + m2 * lc2) * dq1 + (-0.2e1 * m3 * lc3 * sin(q1) * cos(q1 + q3) + 0.2e1 * m3 * lc3 * cos(q1) * sin(q1 + q3)) * dq3 / 0.2e1 0 (-0.2e1 * m3 * lc3 * sin(q1) * cos(q1 + q3) + 0.2e1 * m3 * lc3 * cos(q1) * sin(q1 + q3)) * dq1 / 0.2e1 + (-m3 * lc3 * sin(q1) * cos(q1 + q3) + m3 * lc3 * cos(q1) * sin(q1 + q3)) * dq3; (m3 * lc3 * cos(q1) * q2 * cos(q1 + q3) + m3 * lc3 * sin(q1) * q2 * sin(q1 + q3)) * dq1 + (0.2e1 * m3 * lc3 * sin(q1) * cos(q1 + q3) - 0.2e1 * m3 * lc3 * cos(q1) * sin(q1 + q3)) * dq2 / 0.2e1 (0.2e1 * m3 * lc3 * sin(q1) * cos(q1 + q3) - 0.2e1 * m3 * lc3 * cos(q1) * sin(q1 + q3)) * dq1 / 0.2e1 0;];
% Inertia matrix
M = [0.2e1 * m3 * lc3 * cos(q1 + q3) * sin(q1) * q2 - 0.2e1 * m3 * lc3 * sin(q1 + q3) * cos(q1) * q2 + (m2 + m3) * q2 ^ 2 - 0.2e1 * m2 * lc2 * q2 + m1 * lc1 ^ 2 + In1yy + m2 * lc2 ^ 2 + In3zz + In2zz + m3 * lc3 ^ 2 -m3 * lc3 * sin(q1) * sin(q1 + q3) - m3 * lc3 * cos(q1) * cos(q1 + q3) m3 * lc3 ^ 2 - m3 * lc3 * sin(q1 + q3) * cos(q1) * q2 + m3 * lc3 * cos(q1 + q3) * sin(q1) * q2 + In3zz; -m3 * lc3 * sin(q1) * sin(q1 + q3) - m3 * lc3 * cos(q1) * cos(q1 + q3) m2 + m3 -m3 * lc3 * sin(q1) * sin(q1 + q3) - m3 * lc3 * cos(q1) * cos(q1 + q3); m3 * lc3 ^ 2 - m3 * lc3 * sin(q1 + q3) * cos(q1) * q2 + m3 * lc3 * cos(q1 + q3) * sin(q1) * q2 + In3zz -m3 * lc3 * sin(q1) * sin(q1 + q3) - m3 * lc3 * cos(q1) * cos(q1 + q3) m3 * lc3 ^ 2 + In3zz;];

end

== matlab function model8/RPR   1/Centrifucal and Coriolis Matrix ==
  data: q input; C output; dq input
function C = centriCori(q,dq)
%% Parameters
% Global variables in MATLAB if preferred (remove comments in that case)
% global m1 m2 m3;            % Masses
% global l1 l2 l3;            % Link lengths
% global lc1 lc2 lc3; 	      % Centers of mass
% global In1yy In2zz In3zz;   % Moment of inertia
q1 = q(1);
q2 = q(2);
q3 = q(3);
dq1 = dq(1);
dq2 = dq(2);
dq3 = dq(3);

%syms q1 q2 q3 dq1 dq2 dq3;
m1 = 5; m2 = 5; m3 = 5;
l1 = 0.5; l2 = 0.5; l3 = 0.5;
lc1 = 0.5/2; lc2 = -0.5/2; lc3 = 0.5/2;
In1yy = 1/12*(m1*(l1)^2);
In2zz = 1/12*(m2*(l2)^2);
In3zz = 1/12*(m3*(l3)^2);
gy =9.81;
%% Matrices
% (8.21) Page 295 in book: M(q)*DDq + C(q,Dq)*Dq + G(q) = u
% gy = 9.81
% Gravity vector
%G = [(m3 * cos(q1 + q3) * lc3 + sin(q1) * q2 * m2 + sin(q1) * q2 * m3 + sin(q1) * lc1 * m1 - sin(q1) * m2 * lc2) * gy; -(m2 + m3) * cos(q1) * gy; m3 * cos(q1 + q3) * lc3 * gy;];
% Centrifugal and Coriolis matrix
C = [(-0.2e1 * m3 * lc3 * cos(q1) * sin(q1 + q3) + 0.2e1 * m3 * lc3 * sin(q1) * cos(q1 + q3) + 0.2e1 * (m2 + m3) * q2 - 0.2e1 * m2 * lc2) * dq2 / 0.2e1 + (-0.2e1 * m3 * lc3 * cos(q1) * q2 * cos(q1 + q3) - 0.2e1 * m3 * lc3 * sin(q1) * q2 * sin(q1 + q3)) * dq3 / 0.2e1 (-0.2e1 * m3 * lc3 * cos(q1) * sin(q1 + q3) + 0.2e1 * m3 * lc3 * sin(q1) * cos(q1 + q3) + 0.2e1 * (m2 + m3) * q2 - 0.2e1 * m2 * lc2) * dq1 / 0.2e1 (-0.2e1 * m3 * lc3 * cos(q1) * q2 * cos(q1 + q3) - 0.2e1 * m3 * lc3 * sin(q1) * q2 * sin(q1 + q3)) * dq1 / 0.2e1 + (-m3 * lc3 * cos(q1) * q2 * cos(q1 + q3) - m3 * lc3 * sin(q1) * q2 * sin(q1 + q3)) * dq3; (-m3 * lc3 * sin(q1) * cos(q1 + q3) + m3 * lc3 * cos(q1) * sin(q1 + q3) - (m2 + m3) * q2 + m2 * lc2) * dq1 + (-0.2e1 * m3 * lc3 * sin(q1) * cos(q1 + q3) + 0.2e1 * m3 * lc3 * cos(q1) * sin(q1 + q3)) * dq3 / 0.2e1 0 (-0.2e1 * m3 * lc3 * sin(q1) * cos(q1 + q3) + 0.2e1 * m3 * lc3 * cos(q1) * sin(q1 + q3)) * dq1 / 0.2e1 + (-m3 * lc3 * sin(q1) * cos(q1 + q3) + m3 * lc3 * cos(q1) * sin(q1 + q3)) * dq3; (m3 * lc3 * cos(q1) * q2 * cos(q1 + q3) + m3 * lc3 * sin(q1) * q2 * sin(q1 + q3)) * dq1 + (0.2e1 * m3 * lc3 * sin(q1) * cos(q1 + q3) - 0.2e1 * m3 * lc3 * cos(q1) * sin(q1 + q3)) * dq2 / 0.2e1 (0.2e1 * m3 * lc3 * sin(q1) * cos(q1 + q3) - 0.2e1 * m3 * lc3 * cos(q1) * sin(q1 + q3)) * dq1 / 0.2e1 0;];
% Inertia matrix
%M = [0.2e1 * m3 * lc3 * cos(q1 + q3) * sin(q1) * q2 - 0.2e1 * m3 * lc3 * sin(q1 + q3) * cos(q1) * q2 + (m2 + m3) * q2 ^ 2 - 0.2e1 * m2 * lc2 * q2 + m1 * lc1 ^ 2 + In1yy + m2 * lc2 ^ 2 + In3zz + In2zz + m3 * lc3 ^ 2 -m3 * lc3 * sin(q1) * sin(q1 + q3) - m3 * lc3 * cos(q1) * cos(q1 + q3) m3 * lc3 ^ 2 - m3 * lc3 * sin(q1 + q3) * cos(q1) * q2 + m3 * lc3 * cos(q1 + q3) * sin(q1) * q2 + In3zz; -m3 * lc3 * sin(q1) * sin(q1 + q3) - m3 * lc3 * cos(q1) * cos(q1 + q3) m2 + m3 -m3 * lc3 * sin(q1) * sin(q1 + q3) - m3 * lc3 * cos(q1) * cos(q1 + q3); m3 * lc3 ^ 2 - m3 * lc3 * sin(q1 + q3) * cos(q1) * q2 + m3 * lc3 * cos(q1 + q3) * sin(q1) * q2 + In3zz -m3 * lc3 * sin(q1) * sin(q1 + q3) - m3 * lc3 * cos(q1) * cos(q1 + q3) m3 * lc3 ^ 2 + In3zz;];
end

== matlab function model8/RPR   1/Gravity matrix ==
  data: q input; G output
function G = gravity(q)
%syms q1 q2 q3 dq1 dq2 dq3;
q1 = q(1);
q2 = q(2);
q3 = q(3);

m1 = 5; m2 = 5; m3 = 5;
l1 = 0.5; l2 = 0.5; l3 = 0.5;
lc1 = 0.5/2; lc2 = -0.5/2; lc3 = 0.5/2;
In1yy = 1/12*(m1*(l1)^2);
In2zz = 1/12*(m2*(l2)^2);
In3zz = 1/12*(m3*(l3)^2);
gy = 9.81;
%% Matrices
% (8.21) Page 295 in book: M(q)*DDq + C(q,Dq)*Dq + G(q) = u
% Gravity vector
G = [(m3 * cos(q1 + q3) * lc3 + sin(q1) * q2 * m2 + sin(q1) * q2 * m3 + sin(q1) * lc1 * m1 - sin(q1) * m2 * lc2) * gy; -(m2 + m3) * cos(q1) * gy; m3 * cos(q1 + q3) * lc3 * gy;];

== matlab function model8/RPR   1/Inertia matrix ==
  data: q input; M output
function M = inertia(q)
%% Parameters
% Global variables in MATLAB if preferred (remove comments in that case)
% global m1 m2 m3;            % Masses
% global l1 l2 l3;            % Link lengths
% global lc1 lc2 lc3; 	      % Centers of mass
% global In1yy In2zz In3zz;   % Moment of inertia
q1 = q(1);
q2 = q(2);
q3 = q(3);
%dq1 = dq(1);
%dq2 = dq(2);
%dq3 = dq(3);

%syms q1 q2 q3 dq1 dq2 dq3;
m1 = 5; m2 = 5; m3 = 5;
l1 = 0.5; l2 = 0.5; l3 = 0.5;
lc1 = 0.5/2; lc2 = -0.5/2; lc3 = 0.5/2;
In1yy = 1/12*(m1*(l1)^2);
In2zz = 1/12*(m2*(l2)^2);
In3zz = 1/12*(m3*(l3)^2);
gy =9.81;
%% Matrices
% (8.21) Page 295 in book: M(q)*DDq + C(q,Dq)*Dq + G(q) = u
% gy = 9.81
% Gravity vector
%G = [(m3 * cos(q1 + q3) * lc3 + sin(q1) * q2 * m2 + sin(q1) * q2 * m3 + sin(q1) * lc1 * m1 - sin(q1) * m2 * lc2) * gy; -(m2 + m3) * cos(q1) * gy; m3 * cos(q1 + q3) * lc3 * gy;];
% Centrifugal and Coriolis matrix
%C = [(-0.2e1 * m3 * lc3 * cos(q1) * sin(q1 + q3) + 0.2e1 * m3 * lc3 * sin(q1) * cos(q1 + q3) + 0.2e1 * (m2 + m3) * q2 - 0.2e1 * m2 * lc2) * dq2 / 0.2e1 + (-0.2e1 * m3 * lc3 * cos(q1) * q2 * cos(q1 + q3) - 0.2e1 * m3 * lc3 * sin(q1) * q2 * sin(q1 + q3)) * dq3 / 0.2e1 (-0.2e1 * m3 * lc3 * cos(q1) * sin(q1 + q3) + 0.2e1 * m3 * lc3 * sin(q1) * cos(q1 + q3) + 0.2e1 * (m2 + m3) * q2 - 0.2e1 * m2 * lc2) * dq1 / 0.2e1 (-0.2e1 * m3 * lc3 * cos(q1) * q2 * cos(q1 + q3) - 0.2e1 * m3 * lc3 * sin(q1) * q2 * sin(q1 + q3)) * dq1 / 0.2e1 + (-m3 * lc3 * cos(q1) * q2 * cos(q1 + q3) - m3 * lc3 * sin(q1) * q2 * sin(q1 + q3)) * dq3; (-m3 * lc3 * sin(q1) * cos(q1 + q3) + m3 * lc3 * cos(q1) * sin(q1 + q3) - (m2 + m3) * q2 + m2 * lc2) * dq1 + (-0.2e1 * m3 * lc3 * sin(q1) * cos(q1 + q3) + 0.2e1 * m3 * lc3 * cos(q1) * sin(q1 + q3)) * dq3 / 0.2e1 0 (-0.2e1 * m3 * lc3 * sin(q1) * cos(q1 + q3) + 0.2e1 * m3 * lc3 * cos(q1) * sin(q1 + q3)) * dq1 / 0.2e1 + (-m3 * lc3 * sin(q1) * cos(q1 + q3) + m3 * lc3 * cos(q1) * sin(q1 + q3)) * dq3; (m3 * lc3 * cos(q1) * q2 * cos(q1 + q3) + m3 * lc3 * sin(q1) * q2 * sin(q1 + q3)) * dq1 + (0.2e1 * m3 * lc3 * sin(q1) * cos(q1 + q3) - 0.2e1 * m3 * lc3 * cos(q1) * sin(q1 + q3)) * dq2 / 0.2e1 (0.2e1 * m3 * lc3 * sin(q1) * cos(q1 + q3) - 0.2e1 * m3 * lc3 * cos(q1) * sin(q1 + q3)) * dq1 / 0.2e1 0;];
% Inertia matrix
M = [0.2e1 * m3 * lc3 * cos(q1 + q3) * sin(q1) * q2 - 0.2e1 * m3 * lc3 * sin(q1 + q3) * cos(q1) * q2 + (m2 + m3) * q2 ^ 2 - 0.2e1 * m2 * lc2 * q2 + m1 * lc1 ^ 2 + In1yy + m2 * lc2 ^ 2 + In3zz + In2zz + m3 * lc3 ^ 2 -m3 * lc3 * sin(q1) * sin(q1 + q3) - m3 * lc3 * cos(q1) * cos(q1 + q3) m3 * lc3 ^ 2 - m3 * lc3 * sin(q1 + q3) * cos(q1) * q2 + m3 * lc3 * cos(q1 + q3) * sin(q1) * q2 + In3zz; -m3 * lc3 * sin(q1) * sin(q1 + q3) - m3 * lc3 * cos(q1) * cos(q1 + q3) m2 + m3 -m3 * lc3 * sin(q1) * sin(q1 + q3) - m3 * lc3 * cos(q1) * cos(q1 + q3); m3 * lc3 ^ 2 - m3 * lc3 * sin(q1 + q3) * cos(q1) * q2 + m3 * lc3 * cos(q1 + q3) * sin(q1) * q2 + In3zz -m3 * lc3 * sin(q1) * sin(q1 + q3) - m3 * lc3 * cos(q1) * cos(q1 + q3) m3 * lc3 ^ 2 + In3zz;];

end

== matlab function model8/Link to Task ==
  data: q input; coord output
function coord = fcn(q)
%#codegen
q1 = q(1);
q2 = q(2);
q3 = q(3);

l1 = 0.5; 
l2 = 0.5; 
l3 = 0.5;

coord = [...
            (l2 + l1 + q2) * cos(q1) + l3 * cos(q1 + q3);
            (l2 + l1 + q2) * sin(q1) + l3 * sin(q1 + q3);
            0;
            (l2 + l1 + q2) * cos(q1);
            (l2 + l1 + q2) * sin(q1);
            0;
            l1 * cos(q1);
            l1 * sin(q1);
            0;
        ];

== matlab function model8/Task to Link ==
  data: q output; coord input; q_in input; time input
function q = fcn(coord, q_in, time)
%#codegen
x = coord(1);
y = coord(2);
z = coord(3);

q2 = q_in(2);

l1 = 0.5; 
l2 = 0.5; 
l3 = 0.5;

link_3_fix = pi/2 * cos(time*.5 + pi/2);
ang_link2to3 = atan2(l3*sin(link_3_fix), l1+l2+q2+l3*cos(link_3_fix));
link1_ang  = atan2(y, x) - ang_link2to3;
link2_disp = sqrt(x^2 + y^2)*cos(ang_link2to3) - (l1 + l2 + l3*cos(link_3_fix)); 


q = [...
            link1_ang;
            link2_disp;   
            link_3_fix;                                  % Fixing last joint
        ];

== matlab function model8/Link to Task1 ==
  data: q input; coord output
function coord = fcn(q)
%#codegen
q1 = q(1);
q2 = q(2);
q3 = q(3);

l1 = 0.5; 
l2 = 0.5; 
l3 = 0.5;

coord = [...
            (l2 + l1 + q2) * cos(q1) + l3 * cos(q1 + q3);
            (l2 + l1 + q2) * sin(q1) + l3 * sin(q1 + q3);
            0;
            (l2 + l1 + q2) * cos(q1);
            (l2 + l1 + q2) * sin(q1);
            0;
            l1 * cos(q1);
            l1 * sin(q1);
            0;
        ];
